simulink model "mpc_inertia_mass"  (R2022a)
settings: Solver=daessc  StartTime=0.0  StopTime=simlength  FixedStep=tcontrol  MaxStep=ts  RelTol=1e-3
undefined symbols (not defined in the file): Ad, Aled, Bd, Bled, C, Cle, Fmpc, Gmpc, Kd, Kmpc, Lled, load_torque, simlength, tc, tcontrol
libraries: nesl_utility x17, fl_lib x12, mass_spring_mass_lib x3
settings Model: SimulationMode=accelerator  Creator=dbagn  LastModifiedBy=dabagnara
settings SolverCC: AlgebraicLoopSolver=TrustRegion
settings DataIOCC: ReturnWorkspaceOutputs=off
settings DebuggingCC: UnconnectedInputMsg=warning  UnconnectedOutputMsg=warning  UnconnectedLineMsg=warning  SFMachineParentedDataDiag=warning
settings RTWCC: DLArmComputeVersion=19.05

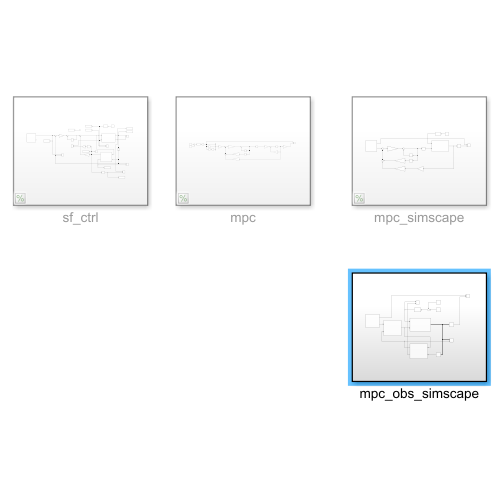
[thumbnail: Simulink's stored preview of the top-level diagram]
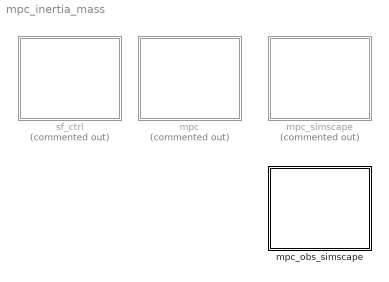
== system mpc_inertia_mass ==
  mpc : Subsystem  Commented=on
  mpc_obs_simscape : Subsystem
  mpc_simscape : Subsystem  Commented=on
  sf_ctrl : Subsystem  Commented=on

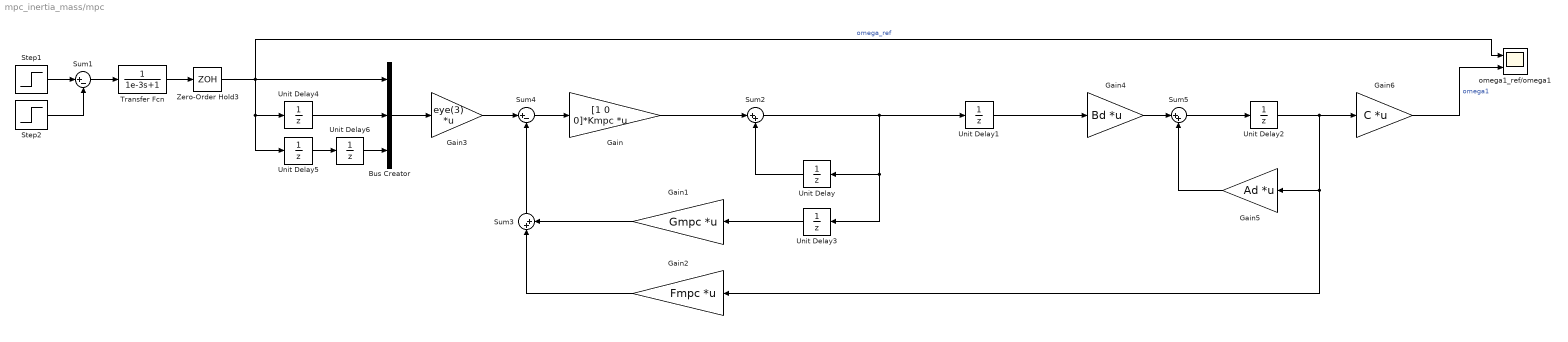
== system mpc_inertia_mass/mpc ==
  Bus Creator : BusCreator  Inputs=3
  Gain : Gain  Gain=[1 0 0]*Kmpc  Multiplication=Matrix(K*u)
  Gain1 : Gain  Gain=Gmpc  Multiplication=Matrix(K*u)
  Gain2 : Gain  Gain=Fmpc  Multiplication=Matrix(K*u)
  Gain3 : Gain  Gain=eye(3)  Multiplication=Matrix(K*u)
  Gain4 : Gain  Gain=Bd  Multiplication=Matrix(K*u)
  Gain5 : Gain  Gain=Ad  Multiplication=Matrix(K*u)
  Gain6 : Gain  Gain=C  Multiplication=Matrix(K*u)
  Step1 : Step  Time=0.2  SampleTime=0
  Step2 : Step  Time=simlength/2  SampleTime=0
  Sum1 : Sum  Inputs=|+-
  Sum2 : Sum  Inputs=|++
  Sum3 : Sum  Inputs=|++
  Sum4 : Sum  Inputs=|+-
  Sum5 : Sum  Inputs=|++
  Transfer Fcn : TransferFcn  Denominator=[1e-3 1]
  Unit Delay{,1..6} (7 alike) : UnitDelay  SampleTime=tcontrol  HasFrameUpgradeWarning=on
  Zero-Order Hold3 : ZeroOrderHold  SampleTime=tcontrol
  omega1_ref/omega1 : Scope  NumInputPorts=2
  wires:
  Step1/1 -> Sum1/1
  Step2/1 -> Sum1/2
  Gain/1 -> Sum2/1
  Unit Delay/1 -> Sum2/2
  Sum4/1 -> Gain/1
  Gain1/1 -> Sum3/2
  Sum3/1 -> Sum4/2
  Gain2/1 -> Sum3/1
  Gain4/1 -> Sum5/1
  Sum5/1 -> Unit Delay2/1
  Gain5/1 -> Sum5/2
  Gain6/1 -> omega1_ref/omega1/2  "omega1"
  Sum1/1 -> Transfer Fcn/1
  Transfer Fcn/1 -> Zero-Order Hold3/1
  Unit Delay3/1 -> Gain1/1
  Unit Delay2/1 -> Gain6/1, Gain2/1, Gain5/1
  Unit Delay5/1 -> Unit Delay6/1
  Unit Delay6/1 -> Bus Creator/3
  Unit Delay4/1 -> Bus Creator/2
  Zero-Order Hold3/1 -> Bus Creator/1, omega1_ref/omega1/1, Unit Delay5/1, Unit Delay4/1  "omega_ref"
  Bus Creator/1 -> Gain3/1
  Gain3/1 -> Sum4/1
  Sum2/1 -> Unit Delay1/1, Unit Delay3/1, Unit Delay/1
  Unit Delay1/1 -> Gain4/1

== system mpc_inertia_mass/mpc_obs_simscape ==
  Load_step : Step  Time=simlength/3  After=load_torque  SampleTime=0
  Load_step1 : Step  Time=2*simlength/3  After=-2*load_torque  SampleTime=0
  Selector : Selector  InputPortWidth=3  IndexOptions=Index vector (dialog)  Indices=[1 2]  OutputSizes=1
  Selector1 : Selector  InputPortWidth=3  IndexOptions=Index vector (dialog)  Indices=1  OutputSizes=1
  Sum : Sum  Inputs=++|
  Transfer Fcn : TransferFcn  Denominator=[1e-1 1]
  mpc : Subsystem
  observer td : Subsystem
  omega1_ref/omega1 : Scope  NumInputPorts=2
  omega1_ref/omega2 : Scope  NumInputPorts=2
  rference generator : Subsystem
  "simscape_plant " : Subsystem
  tau2/tau2_hat : Scope  NumInputPorts=2
  wires:
  Transfer Fcn/1 -> tau2/tau2_hat/1, "simscape_plant "/1(tau2)  "tau_2_flt"
  rference generator/1(omega_ref) -> omega1_ref/omega1/1
  "simscape_plant "/1(state) -> omega1_ref/omega2/1, Selector1/1, Selector/1  "omega1"
  Selector/1 -> omega1_ref/omega1/2  "omega12"
  Selector1/1 -> observer td/2(y)
  observer td/1(x_hat) -> omega1_ref/omega2/2, mpc/2(x_hat)
  observer td/2(tau2_hat) -> tau2/tau2_hat/2
  mpc/1(tau1) -> "simscape_plant "/2(tau1), observer td/1(u)
  rference generator/2(omega_ref_stack) -> mpc/1(yref)
  Load_step/1 -> Sum/2  "tau_2"
  Sum/1 -> Transfer Fcn/1
  Load_step1/1 -> Sum/1  "tau_2"

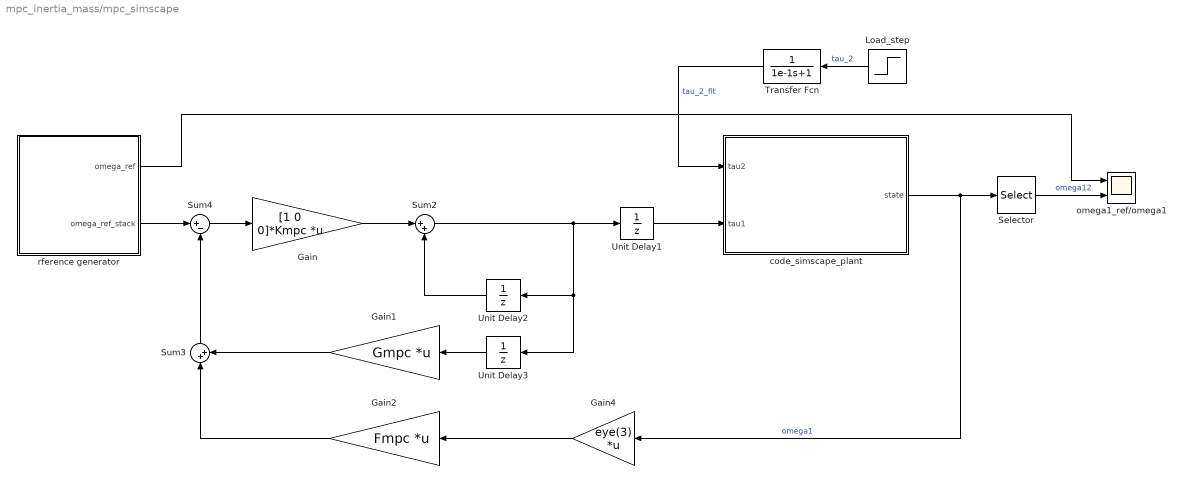
== system mpc_inertia_mass/mpc_simscape ==
  Gain : Gain  Gain=[1 0 0]*Kmpc  Multiplication=Matrix(K*u)
  Gain1 : Gain  Gain=Gmpc  Multiplication=Matrix(K*u)
  Gain2 : Gain  Gain=Fmpc  Multiplication=Matrix(K*u)
  Gain4 : Gain  Gain=eye(3)  Multiplication=Matrix(K*u)
  Load_step : Step  Time=simlength/3  After=load_torque  SampleTime=0
  Selector : Selector  InputPortWidth=3  IndexOptions=Index vector (dialog)  Indices=[1 2]  OutputSizes=1
  Sum2 : Sum  Inputs=|++
  Sum3 : Sum  Inputs=|++
  Sum4 : Sum  Inputs=|+-
  Transfer Fcn : TransferFcn  Denominator=[1e-1 1]
  Unit Delay1 : UnitDelay  SampleTime=tcontrol  HasFrameUpgradeWarning=on
  Unit Delay2 : UnitDelay  SampleTime=tcontrol  HasFrameUpgradeWarning=on
  Unit Delay3 : UnitDelay  SampleTime=tcontrol  HasFrameUpgradeWarning=on
  "code_simscape_plant " : Subsystem
  omega1_ref/omega1 : Scope  NumInputPorts=2
  rference generator : Subsystem
  wires:
  Selector/1 -> omega1_ref/omega1/2  "omega12"
  Gain2/1 -> Sum3/1
  Sum3/1 -> Sum4/2
  Gain1/1 -> Sum3/2
  Sum4/1 -> Gain/1
  Gain/1 -> Sum2/1
  "code_simscape_plant "/1(state) -> Selector/1, Gain4/1  "omega1"
  Gain4/1 -> Gain2/1
  Unit Delay2/1 -> Sum2/2
  Unit Delay3/1 -> Gain1/1
  Sum2/1 -> Unit Delay1/1, Unit Delay3/1, Unit Delay2/1
  Unit Delay1/1 -> "code_simscape_plant "/2(tau1)
  rference generator/1(omega_ref) -> omega1_ref/omega1/1
  rference generator/2(omega_ref_stack) -> Sum4/1
  Load_step/1 -> Transfer Fcn/1  "tau_2"
  Transfer Fcn/1 -> "code_simscape_plant "/1(tau2)  "tau_2_flt"

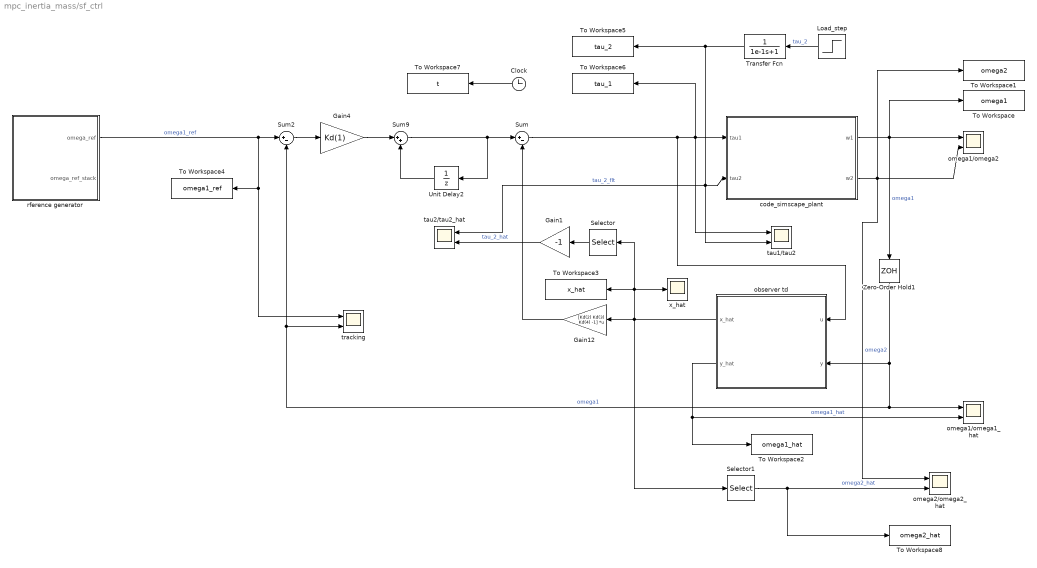
== system mpc_inertia_mass/sf_ctrl ==
  Clock : Clock
  Gain1 : Gain  Gain=-1
  Gain12 : Gain  Gain=[Kd(2) Kd(3) Kd(4) -1]  Multiplication=Matrix(K*u)
  Gain4 : Gain  Gain=Kd(1)
  Load_step : Step  Time=simlength/3  After=load_torque  SampleTime=0
  Selector : Selector  InputPortWidth=4  IndexOptions=Index vector (dialog)  Indices=4  OutputSizes=1
  Selector1 : Selector  InputPortWidth=4  IndexOptions=Index vector (dialog)  Indices=2  OutputSizes=1
  Sum : Sum  Inputs=|+-
  Sum2 : Sum  Inputs=|+-
  Sum9 : Sum  Inputs=|++
  To Workspace : ToWorkspace  VariableName=omega1  SampleTime=tc
      settings: MaxDataPoints=Nc
  To Workspace1 : ToWorkspace  VariableName=omega2  SampleTime=tc
      settings: MaxDataPoints=Nc
  To Workspace2 : ToWorkspace  VariableName=omega1_hat  SampleTime=tc
      settings: MaxDataPoints=Nc
  To Workspace3 : ToWorkspace  VariableName=x_hat  SampleTime=tc
      settings: MaxDataPoints=Nc
  To Workspace4 : ToWorkspace  VariableName=omega1_ref  SampleTime=tc
      settings: MaxDataPoints=Nc
  To Workspace5 : ToWorkspace  VariableName=tau_2  SampleTime=tc
      settings: MaxDataPoints=Nc
  To Workspace6 : ToWorkspace  VariableName=tau_1  SampleTime=tc
      settings: MaxDataPoints=Nc
  To Workspace7 : ToWorkspace  VariableName=t  SampleTime=tc
      settings: MaxDataPoints=Nc
  To Workspace8 : ToWorkspace  VariableName=omega2_hat  SampleTime=tc
      settings: MaxDataPoints=Nc
  Transfer Fcn : TransferFcn  Denominator=[1e-1 1]
  Unit Delay2 : UnitDelay  SampleTime=tcontrol  HasFrameUpgradeWarning=on
  Zero-Order Hold1 : ZeroOrderHold  SampleTime=tcontrol
  "code_simscape_plant " : Subsystem
  observer td : Subsystem
  omega1/omega1_hat : Scope  NumInputPorts=2
  omega1/omega2 : Scope  NumInputPorts=2
  omega2/omega2_hat : Scope  NumInputPorts=2
  rference generator : Subsystem
  tau1/tau2 : Scope  NumInputPorts=2
  tau2/tau2_hat : Scope  NumInputPorts=2
  tracking : Scope  NumInputPorts=2
  x_hat : Scope
  wires:
  Sum9/1 -> Sum/1, Unit Delay2/1
  Transfer Fcn/1 -> To Workspace5/1, "code_simscape_plant "/2(tau2), tau1/tau2/2, tau2/tau2_hat/1  "tau_2_flt"
  observer td/1(x_hat) -> Selector1/1, Selector/1, To Workspace3/1, x_hat/1, Gain12/1
  Selector1/1 -> To Workspace8/1, omega2/omega2_hat/2  "omega2_hat"
  Gain12/1 -> Sum/2
  "code_simscape_plant "/2(w2) -> To Workspace1/1, omega1/omega2/2, omega2/omega2_hat/1  "omega2"
  "code_simscape_plant "/1(w1) -> Zero-Order Hold1/1, To Workspace/1, omega1/omega2/1  "omega1"
  Gain4/1 -> Sum9/1
  Zero-Order Hold1/1 -> tracking/2, Sum2/2, omega1/omega1_hat/1, observer td/2(y)  "omega1"
  Load_step/1 -> Transfer Fcn/1  "tau_2"
  observer td/2(y_hat) -> To Workspace2/1, omega1/omega1_hat/2  "omega1_hat"
  rference generator/1(omega_ref) -> To Workspace4/1, tracking/1, Sum2/1  "omega1_ref"
  Gain1/1 -> tau2/tau2_hat/2  "tau_2_hat"
  Clock/1 -> To Workspace7/1
  Sum2/1 -> Gain4/1
  Selector/1 -> Gain1/1
  Unit Delay2/1 -> Sum9/2
  Sum/1 -> tau1/tau2/1, "code_simscape_plant "/1(tau1), To Workspace6/1, observer td/1(u)

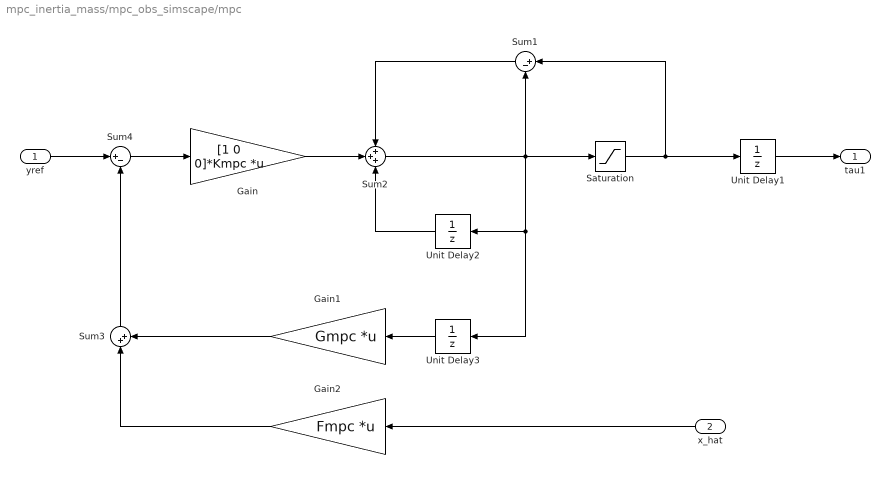
== system mpc_inertia_mass/mpc_obs_simscape/mpc ==
  yref : Inport
  x_hat : Inport  Port=2
  Gain : Gain  Gain=[1 0 0]*Kmpc  Multiplication=Matrix(K*u)
  Gain1 : Gain  Gain=Gmpc  Multiplication=Matrix(K*u)
  Gain2 : Gain  Gain=Fmpc  Multiplication=Matrix(K*u)
  Saturation : Saturate  UpperLimit=2000  LowerLimit=-2000
  Sum1 : Sum  Inputs=|+-
  Sum2 : Sum  Inputs=+++
  Sum3 : Sum  Inputs=|++
  Sum4 : Sum  Inputs=|+-
  Unit Delay1 : UnitDelay  SampleTime=tcontrol  HasFrameUpgradeWarning=on
  Unit Delay2 : UnitDelay  SampleTime=tcontrol  HasFrameUpgradeWarning=on
  Unit Delay3 : UnitDelay  SampleTime=tcontrol  HasFrameUpgradeWarning=on
  tau1 : Outport
  wires:
  Sum3/1 -> Sum4/2
  Gain1/1 -> Sum3/2
  Sum4/1 -> Gain/1
  Gain2/1 -> Sum3/1
  x_hat/1 -> Gain2/1
  Unit Delay3/1 -> Gain1/1
  yref/1 -> Sum4/1
  Sum2/1 -> Sum1/2, Saturation/1, Unit Delay2/1, Unit Delay3/1
  Gain/1 -> Sum2/2
  Unit Delay2/1 -> Sum2/3
  Sum1/1 -> Sum2/1
  Saturation/1 -> Unit Delay1/1, Sum1/1
  Unit Delay1/1 -> tau1/1

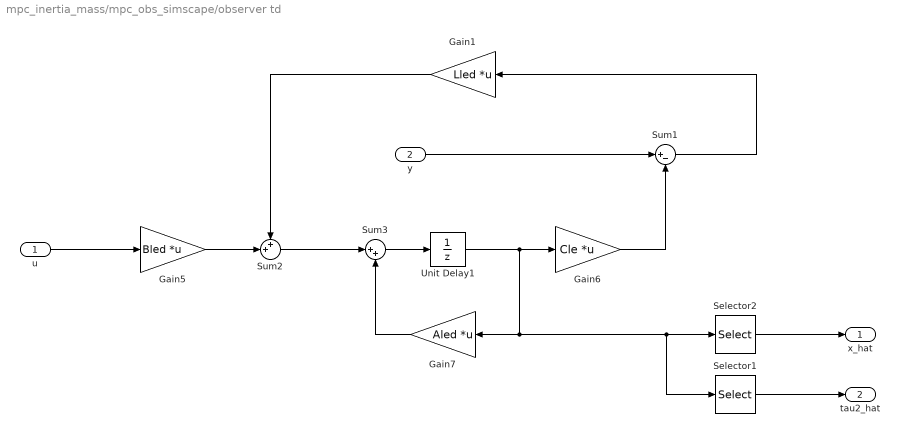
== system mpc_inertia_mass/mpc_obs_simscape/observer td ==
  u : Inport
  y : Inport  Port=2
  Gain1 : Gain  Gain=Lled  Multiplication=Matrix(K*u)
  Gain5 : Gain  Gain=Bled  Multiplication=Matrix(K*u)
  Gain6 : Gain  Gain=Cle  Multiplication=Matrix(K*u)
  Gain7 : Gain  Gain=Aled  Multiplication=Matrix(K*u)
  Selector1 : Selector  InputPortWidth=4  IndexOptions=Index vector (dialog)  Indices=4  OutputSizes=1
  Selector2 : Selector  InputPortWidth=4  IndexOptions=Index vector (dialog)  Indices=[1 2 3]  OutputSizes=1
  Sum1 : Sum  Inputs=|+-
  Sum2 : Sum  Inputs=++|
  Sum3 : Sum  Inputs=|++
  Unit Delay1 : UnitDelay  SampleTime=tcontrol  HasFrameUpgradeWarning=on
  x_hat : Outport
  tau2_hat : Outport  Port=2
  wires:
  Sum2/1 -> Sum3/1
  Sum3/1 -> Unit Delay1/1
  Gain7/1 -> Sum3/2
  Gain6/1 -> Sum1/2
  Sum1/1 -> Gain1/1
  u/1 -> Gain5/1
  Gain1/1 -> Sum2/1
  Gain5/1 -> Sum2/2
  Unit Delay1/1 -> Selector1/1, Selector2/1, Gain7/1, Gain6/1
  y/1 -> Sum1/1
  Selector2/1 -> x_hat/1
  Selector1/1 -> tau2_hat/1

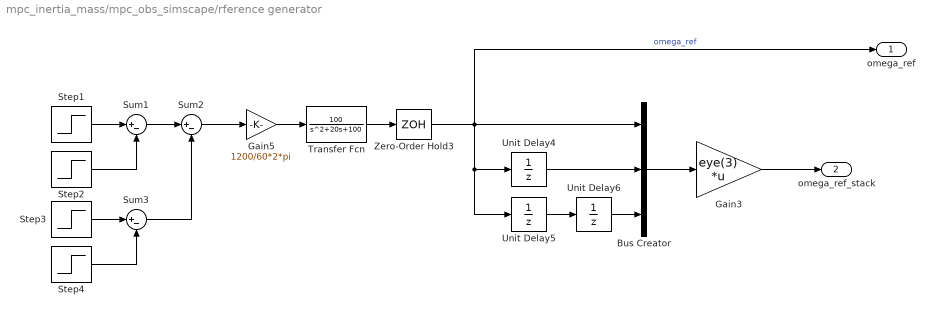
== system mpc_inertia_mass/mpc_obs_simscape/rference generator ==
  Bus Creator : BusCreator  Inputs=3
  Gain3 : Gain  Gain=eye(3)  Multiplication=Matrix(K*u)
  Gain5 : Gain  Gain=1200/60*2*pi
  Step1 : Step  Time=2  SampleTime=0
  Step2 : Step  Time=simlength/4  SampleTime=0
  Step3 : Step  Time=simlength/2  SampleTime=0
  Step4 : Step  Time=2*simlength/3  SampleTime=0
  Sum1 : Sum  Inputs=|+-
  Sum2 : Sum  Inputs=|+-
  Sum3 : Sum  Inputs=|+-
  Transfer Fcn : TransferFcn  Numerator=[100]  Denominator=[1 20 100]
  Unit Delay4 : UnitDelay  SampleTime=tcontrol  HasFrameUpgradeWarning=on
  Unit Delay5 : UnitDelay  SampleTime=tcontrol  HasFrameUpgradeWarning=on
  Unit Delay6 : UnitDelay  SampleTime=tcontrol  HasFrameUpgradeWarning=on
  Zero-Order Hold3 : ZeroOrderHold  SampleTime=tcontrol
  omega_ref : Outport
  omega_ref_stack : Outport  Port=2
  wires:
  Sum3/1 -> Sum2/2
  Step4/1 -> Sum3/2
  Step3/1 -> Sum3/1
  Sum2/1 -> Gain5/1
  Sum1/1 -> Sum2/1
  Gain3/1 -> omega_ref_stack/1
  Step1/1 -> Sum1/1
  Transfer Fcn/1 -> Zero-Order Hold3/1
  Step2/1 -> Sum1/2
  Unit Delay5/1 -> Unit Delay6/1
  Unit Delay6/1 -> Bus Creator/3
  Zero-Order Hold3/1 -> Bus Creator/1, Unit Delay5/1, Unit Delay4/1, omega_ref/1  "omega_ref"
  Bus Creator/1 -> Gain3/1
  Gain5/1 -> Transfer Fcn/1
  Unit Delay4/1 -> Bus Creator/2

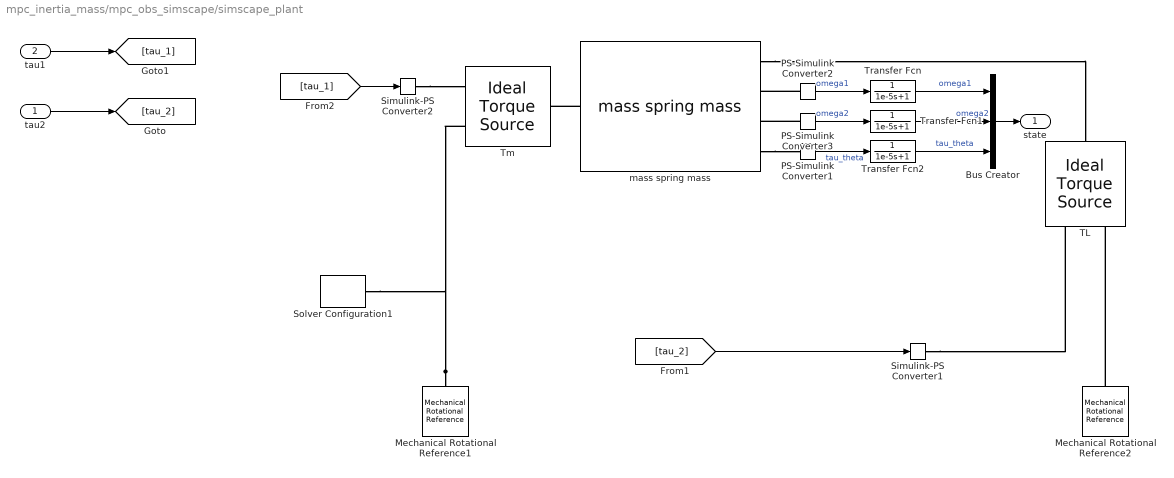
== system mpc_inertia_mass/mpc_obs_simscape/simscape_plant  ==
  tau2 : Inport
  tau1 : Inport  Port=2
  Bus Creator : BusCreator  Inputs=3
  Mechanical Rotational Reference1 : fl_lib/Mechanical/Rotational Elements/Mechanical Rotational Reference
      settings: SourceProductBaseCode=PW,SS,VE
  Mechanical Rotational Reference2 : fl_lib/Mechanical/Rotational Elements/Mechanical Rotational Reference
      settings: SourceProductBaseCode=PW,SS,VE
  PS-Simulink Converter1 : nesl_utility/PS-Simulink Converter  PhysicalDomain=network_engine_domain  SubClassName=ps_output  LeftPortType=input  RightPortType=output  PseudoPeriodic=off  Frequencies=[]  VectorFormat=1-D array  Unit=N*m  AffineConversion=on
      settings: SourceProductBaseCode=SS,PW,VE
  PS-Simulink Converter2 : nesl_utility/PS-Simulink Converter  PhysicalDomain=network_engine_domain  SubClassName=ps_output  LeftPortType=input  RightPortType=output  PseudoPeriodic=off  Frequencies=[]  VectorFormat=1-D array  Unit=rad/s  AffineConversion=on
      settings: SourceProductBaseCode=SS,PW,VE
  PS-Simulink Converter3 : nesl_utility/PS-Simulink Converter  PhysicalDomain=network_engine_domain  SubClassName=ps_output  LeftPortType=input  RightPortType=output  PseudoPeriodic=off  Frequencies=[]  VectorFormat=1-D array  Unit=rad/s  AffineConversion=on
      settings: SourceProductBaseCode=SS,PW,VE
  Simulink-PS Converter1 : nesl_utility/Simulink-PS Converter  PhysicalDomain=network_engine_domain  SubClassName=ps_input  LeftPortType=input  RightPortType=output  PseudoPeriodic=off  Frequencies=[]  NoiseDistribution=none  NoiseParameters=[]  Unit=1  AffineConversion=off  FilteringAndDerivatives=provide  SimscapeFilterOrder=1  InputFilterTimeConstant=0.001  UdotUserProvided=0
      settings: SourceProductBaseCode=SS,PW,VE
  Simulink-PS Converter2 : nesl_utility/Simulink-PS Converter  PhysicalDomain=network_engine_domain  SubClassName=ps_input  LeftPortType=input  RightPortType=output  PseudoPeriodic=off  Frequencies=[]  NoiseDistribution=none  NoiseParameters=[]  Unit=1  AffineConversion=off  FilteringAndDerivatives=provide  SimscapeFilterOrder=1  InputFilterTimeConstant=0.001  UdotUserProvided=0
      settings: SourceProductBaseCode=SS,PW,VE
  Solver Configuration1 : nesl_utility/Solver Configuration  PhysicalDomain=network_engine_domain  SubClassName=solver  LeftPortType=input  RightPortType=generic  Tones=[]  Harmonics=[]  SimulateNoise=off  Profile=off  UseLocalSampling=off  EnableSwitchedLinearOptims=on  FrequencyDomain=off  UseCCode=off  RelTol=0.001  AbsTol=1e-06  MinStep=1e-09  ToWorkspace=off  RevertToSquareIcSolve=off  NumHomotopyIterations=100  PhasorMode=off  PhasorModeNumHarmonics=1  IndexReductionMethod=DerivativeReplacement  DoDC=off  ResidualTolerance=1e-09  UseLocalSolver=on  LocalSolverChoice=NE_BACKWARD_EULER_ADVANCER  LocalSolverSampleTime=ts  DoFixedCost=on  MaxNonlinIter=3  MaxModeIter=2  ComputeImpulses=off  ImpulseIterations=2  LinearAlgebra=auto  LinearAlgebraNumThread=0  EquationFormulation=NE_TIME_EF  DelaysMemoryBudget=1024  AutomaticFiltering=on  FilteringTimeConstant=0.001  PartitionStorageMethod=AS_NEEDED  PartitionMemoryBudget=1024  PartitionMethod=ROBUST
      settings: SourceProductBaseCode=SS,PW,VE
  TL : fl_lib/Mechanical/Mechanical Sources/Ideal Torque Source
      settings: SourceProductBaseCode=PW,SS,VE
  "Tm " : fl_lib/Mechanical/Mechanical Sources/Ideal Torque Source
      settings: SourceProductBaseCode=PW,SS,VE
  Transfer Fcn : TransferFcn  Denominator=[1e-5 1]
  Transfer Fcn1 : TransferFcn  Denominator=[1e-5 1]
  Transfer Fcn2 : TransferFcn  Denominator=[1e-5 1]
  mass spring mass : mass_spring_mass_lib/mass spring mass  b1=b N*m/(rad/s)  J1=J1 kg*m^2  b2=b N*m/(rad/s)  J2=J2 kg*m^2  b_theta=b_theta N*m/(rad/s)  k_theta=k_theta N*m/rad  omega_1_specify=off  omega_1_priority=None  omega_1=0 rad/s  omega_1_nominal_specify=off  omega_1_nominal_unit=rad/s  omega_1_nominal_value=1  omega_2_specify=off  omega_2_priority=None  omega_2=0 rad/s  omega_2_nominal_specify=off  omega_2_nominal_unit=rad/s  omega_2_nominal_value=1  tau_1_specify=off  tau_1_priority=None  tau_1=0 N*m  tau_1_nominal_specify=off  tau_1_nominal_unit=N*m  tau_1_nominal_value=1  tau_2_specify=off  tau_2_priority=None  tau_2=0 N*m  tau_2_nominal_specify=off  tau_2_nominal_unit=N*m  tau_2_nominal_value=1  tau_theta_specify=off  tau_theta_priority=None  tau_theta=0 N*m  tau_theta_nominal_specify=off  tau_theta_nominal_unit=N*m  tau_theta_nominal_value=1
      settings: InternalSimscapePortConfiguration="{\"Bottom\":[],\"Left\":[{\"id\":\"S1\",\"label\":\"S1\",\"type\":\"foundation.mechanical.rotational.rotational\"}],\"Right\":[{\"id\":\"S2\",\"label\":\"S2\",\"type\":\"foundation.mechanical.rotational.rotational\"},{\"id\":\"omega1_out\",\"label\":\"omega1\",\"type\":\"output\"},{\"id\":\"omega2_out\",\"label\":\"omega2\",\"type\":\"output\"},{\"id\":\"tau_theta_out\",\"label\":\"tau_theta\",\"type\":\"output\"}],\"Top\":[]}"
  state : Outport
  wires:
  Transfer Fcn2/1 -> Bus Creator/3  "tau_theta"
  Transfer Fcn1/1 -> Bus Creator/2  "omega2"
  Transfer Fcn/1 -> Bus Creator/1  "omega1"
  PS-Simulink Converter1/1 -> Transfer Fcn2/1  "tau_theta"
  PS-Simulink Converter3/1 -> Transfer Fcn1/1  "omega2"
  PS-Simulink Converter2/1 -> Transfer Fcn/1  "omega1"
  tau2/1 -> [tau_2]
  [tau_1] -> Simulink-PS Converter2/1
  tau1/1 -> [tau_1]
  [tau_2] -> Simulink-PS Converter1/1
  Bus Creator/1 -> state/1
  connections:
  Mechanical Rotational Reference2/LConn1 -- TL/RConn2
  Mechanical Rotational Reference1/LConn1 -- "Tm "/RConn2 -- Solver Configuration1/RConn1
  mass spring mass/RConn1 -- TL/LConn1
  Simulink-PS Converter1/RConn1 -- TL/RConn1
  mass spring mass/LConn1 -- "Tm "/LConn1
  Simulink-PS Converter2/RConn1 -- "Tm "/RConn1
  mass spring mass/RConn4 -- PS-Simulink Converter1/LConn1
  PS-Simulink Converter3/LConn1 -- mass spring mass/RConn3
  PS-Simulink Converter2/LConn1 -- mass spring mass/RConn2

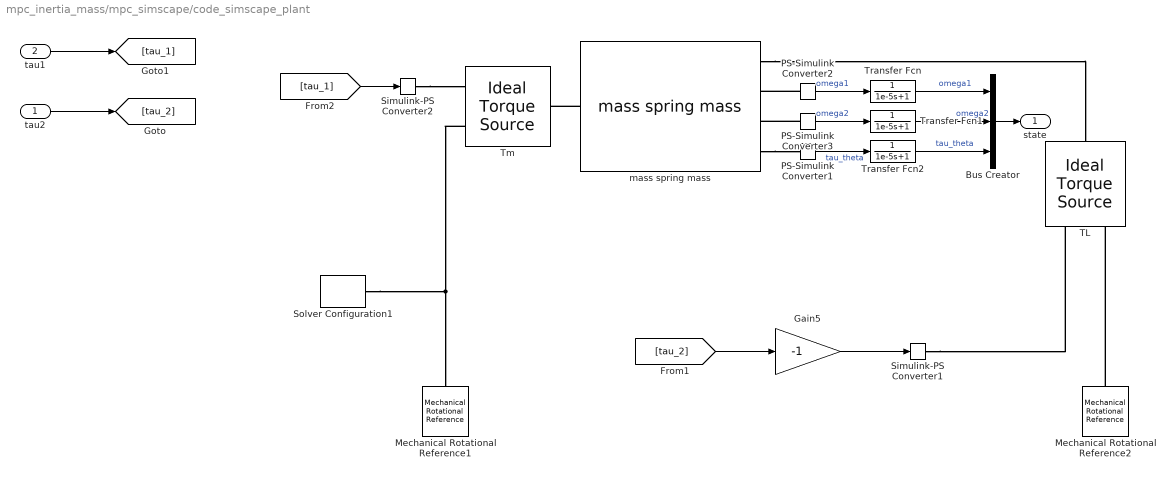
== system mpc_inertia_mass/mpc_simscape/code_simscape_plant  ==
  tau2 : Inport
  tau1 : Inport  Port=2
  Bus Creator : BusCreator  Inputs=3
  Gain5 : Gain  Gain=-1
  Mechanical Rotational Reference1 : fl_lib/Mechanical/Rotational Elements/Mechanical Rotational Reference
      settings: SourceProductBaseCode=PW,SS,VE
  Mechanical Rotational Reference2 : fl_lib/Mechanical/Rotational Elements/Mechanical Rotational Reference
      settings: SourceProductBaseCode=PW,SS,VE
  PS-Simulink Converter1 : nesl_utility/PS-Simulink Converter  PhysicalDomain=network_engine_domain  SubClassName=ps_output  LeftPortType=input  RightPortType=output  PseudoPeriodic=off  Frequencies=[]  VectorFormat=1-D array  Unit=N*m  AffineConversion=on
      settings: SourceProductBaseCode=SS,PW,VE
  PS-Simulink Converter2 : nesl_utility/PS-Simulink Converter  PhysicalDomain=network_engine_domain  SubClassName=ps_output  LeftPortType=input  RightPortType=output  PseudoPeriodic=off  Frequencies=[]  VectorFormat=1-D array  Unit=rad/s  AffineConversion=on
      settings: SourceProductBaseCode=SS,PW,VE
  PS-Simulink Converter3 : nesl_utility/PS-Simulink Converter  PhysicalDomain=network_engine_domain  SubClassName=ps_output  LeftPortType=input  RightPortType=output  PseudoPeriodic=off  Frequencies=[]  VectorFormat=1-D array  Unit=rad/s  AffineConversion=on
      settings: SourceProductBaseCode=SS,PW,VE
  Simulink-PS Converter1 : nesl_utility/Simulink-PS Converter  PhysicalDomain=network_engine_domain  SubClassName=ps_input  LeftPortType=input  RightPortType=output  PseudoPeriodic=off  Frequencies=[]  NoiseDistribution=none  NoiseParameters=[]  Unit=1  AffineConversion=off  FilteringAndDerivatives=provide  SimscapeFilterOrder=1  InputFilterTimeConstant=0.001  UdotUserProvided=0
      settings: SourceProductBaseCode=SS,PW,VE
  Simulink-PS Converter2 : nesl_utility/Simulink-PS Converter  PhysicalDomain=network_engine_domain  SubClassName=ps_input  LeftPortType=input  RightPortType=output  PseudoPeriodic=off  Frequencies=[]  NoiseDistribution=none  NoiseParameters=[]  Unit=1  AffineConversion=off  FilteringAndDerivatives=provide  SimscapeFilterOrder=1  InputFilterTimeConstant=0.001  UdotUserProvided=0
      settings: SourceProductBaseCode=SS,PW,VE
  Solver Configuration1 : nesl_utility/Solver Configuration  PhysicalDomain=network_engine_domain  SubClassName=solver  LeftPortType=input  RightPortType=generic  Tones=[]  Harmonics=[]  SimulateNoise=off  Profile=off  UseLocalSampling=off  EnableSwitchedLinearOptims=on  FrequencyDomain=off  UseCCode=off  RelTol=0.001  AbsTol=1e-06  MinStep=1e-09  ToWorkspace=off  RevertToSquareIcSolve=off  NumHomotopyIterations=100  PhasorMode=off  PhasorModeNumHarmonics=1  IndexReductionMethod=DerivativeReplacement  DoDC=off  ResidualTolerance=1e-09  UseLocalSolver=on  LocalSolverChoice=NE_TRAPEZOIDAL_ADVANCER  LocalSolverSampleTime=ts  DoFixedCost=on  MaxNonlinIter=3  MaxModeIter=2  ComputeImpulses=off  ImpulseIterations=2  LinearAlgebra=auto  LinearAlgebraNumThread=0  EquationFormulation=NE_TIME_EF  DelaysMemoryBudget=1024  AutomaticFiltering=on  FilteringTimeConstant=0.001  PartitionStorageMethod=AS_NEEDED  PartitionMemoryBudget=1024  PartitionMethod=ROBUST
      settings: SourceProductBaseCode=SS,PW,VE
  TL : fl_lib/Mechanical/Mechanical Sources/Ideal Torque Source
      settings: SourceProductBaseCode=PW,SS,VE
  "Tm " : fl_lib/Mechanical/Mechanical Sources/Ideal Torque Source
      settings: SourceProductBaseCode=PW,SS,VE
  Transfer Fcn : TransferFcn  Denominator=[1e-5 1]
  Transfer Fcn1 : TransferFcn  Denominator=[1e-5 1]
  Transfer Fcn2 : TransferFcn  Denominator=[1e-5 1]
  mass spring mass : mass_spring_mass_lib/mass spring mass  b1=b N*m/(rad/s)  J1=J1 kg*m^2  b2=b N*m/(rad/s)  J2=J2 kg*m^2  b_theta=b_theta N*m/(rad/s)  k_theta=k_theta N*m/rad  omega_1_specify=off  omega_1_priority=None  omega_1=0 rad/s  omega_1_nominal_specify=off  omega_1_nominal_unit=rad/s  omega_1_nominal_value=1  omega_2_specify=off  omega_2_priority=None  omega_2=0 rad/s  omega_2_nominal_specify=off  omega_2_nominal_unit=rad/s  omega_2_nominal_value=1  tau_1_specify=off  tau_1_priority=None  tau_1=0 N*m  tau_1_nominal_specify=off  tau_1_nominal_unit=N*m  tau_1_nominal_value=1  tau_2_specify=off  tau_2_priority=None  tau_2=0 N*m  tau_2_nominal_specify=off  tau_2_nominal_unit=N*m  tau_2_nominal_value=1  tau_theta_specify=off  tau_theta_priority=None  tau_theta=0 N*m  tau_theta_nominal_specify=off  tau_theta_nominal_unit=N*m  tau_theta_nominal_value=1
      settings: InternalSimscapePortConfiguration="{\"Bottom\":[],\"Left\":[{\"id\":\"S1\",\"label\":\"S1\",\"type\":\"foundation.mechanical.rotational.rotational\"}],\"Right\":[{\"id\":\"S2\",\"label\":\"S2\",\"type\":\"foundation.mechanical.rotational.rotational\"},{\"id\":\"omega1_out\",\"label\":\"omega1\",\"type\":\"output\"},{\"id\":\"omega2_out\",\"label\":\"omega2\",\"type\":\"output\"},{\"id\":\"tau_theta_out\",\"label\":\"tau_theta\",\"type\":\"output\"}],\"Top\":[]}"
  state : Outport
  wires:
  Bus Creator/1 -> state/1
  Gain5/1 -> Simulink-PS Converter1/1
  tau1/1 -> [tau_1]
  [tau_1] -> Simulink-PS Converter2/1
  tau2/1 -> [tau_2]
  [tau_2] -> Gain5/1
  PS-Simulink Converter2/1 -> Transfer Fcn/1  "omega1"
  PS-Simulink Converter3/1 -> Transfer Fcn1/1  "omega2"
  PS-Simulink Converter1/1 -> Transfer Fcn2/1  "tau_theta"
  Transfer Fcn/1 -> Bus Creator/1  "omega1"
  Transfer Fcn1/1 -> Bus Creator/2  "omega2"
  Transfer Fcn2/1 -> Bus Creator/3  "tau_theta"
  connections:
  PS-Simulink Converter2/LConn1 -- mass spring mass/RConn2
  PS-Simulink Converter3/LConn1 -- mass spring mass/RConn3
  mass spring mass/RConn4 -- PS-Simulink Converter1/LConn1
  Simulink-PS Converter2/RConn1 -- "Tm "/RConn1
  mass spring mass/LConn1 -- "Tm "/LConn1
  Simulink-PS Converter1/RConn1 -- TL/RConn1
  mass spring mass/RConn1 -- TL/LConn1
  Solver Configuration1/RConn1 -- "Tm "/RConn2 -- Mechanical Rotational Reference1/LConn1
  Mechanical Rotational Reference2/LConn1 -- TL/RConn2

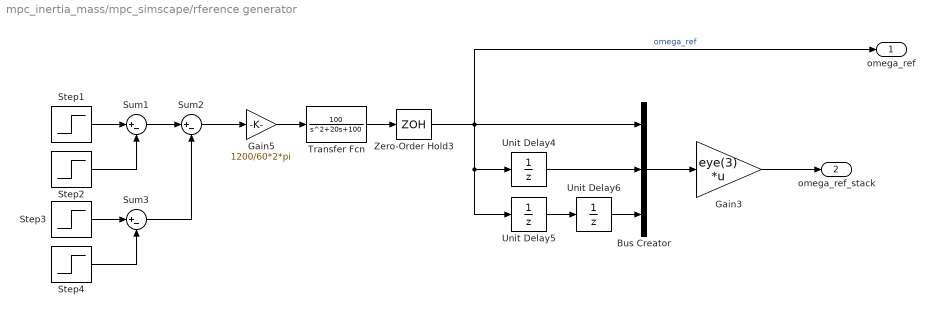
== system mpc_inertia_mass/mpc_simscape/rference generator ==
  Bus Creator : BusCreator  Inputs=3
  Gain3 : Gain  Gain=eye(3)  Multiplication=Matrix(K*u)
  Gain5 : Gain  Gain=1200/60*2*pi
  Step1 : Step  Time=2  SampleTime=0
  Step2 : Step  Time=simlength/4  SampleTime=0
  Step3 : Step  Time=simlength/2  SampleTime=0
  Step4 : Step  Time=2*simlength/3  SampleTime=0
  Sum1 : Sum  Inputs=|+-
  Sum2 : Sum  Inputs=|+-
  Sum3 : Sum  Inputs=|+-
  Transfer Fcn : TransferFcn  Numerator=[100]  Denominator=[1 20 100]
  Unit Delay4 : UnitDelay  SampleTime=tcontrol  HasFrameUpgradeWarning=on
  Unit Delay5 : UnitDelay  SampleTime=tcontrol  HasFrameUpgradeWarning=on
  Unit Delay6 : UnitDelay  SampleTime=tcontrol  HasFrameUpgradeWarning=on
  Zero-Order Hold3 : ZeroOrderHold  SampleTime=tcontrol
  omega_ref : Outport
  omega_ref_stack : Outport  Port=2
  wires:
  Unit Delay4/1 -> Bus Creator/2
  Gain5/1 -> Transfer Fcn/1
  Bus Creator/1 -> Gain3/1
  Zero-Order Hold3/1 -> omega_ref/1, Unit Delay4/1, Unit Delay5/1, Bus Creator/1  "omega_ref"
  Unit Delay6/1 -> Bus Creator/3
  Unit Delay5/1 -> Unit Delay6/1
  Step2/1 -> Sum1/2
  Transfer Fcn/1 -> Zero-Order Hold3/1
  Step1/1 -> Sum1/1
  Gain3/1 -> omega_ref_stack/1
  Sum1/1 -> Sum2/1
  Sum2/1 -> Gain5/1
  Step3/1 -> Sum3/1
  Step4/1 -> Sum3/2
  Sum3/1 -> Sum2/2

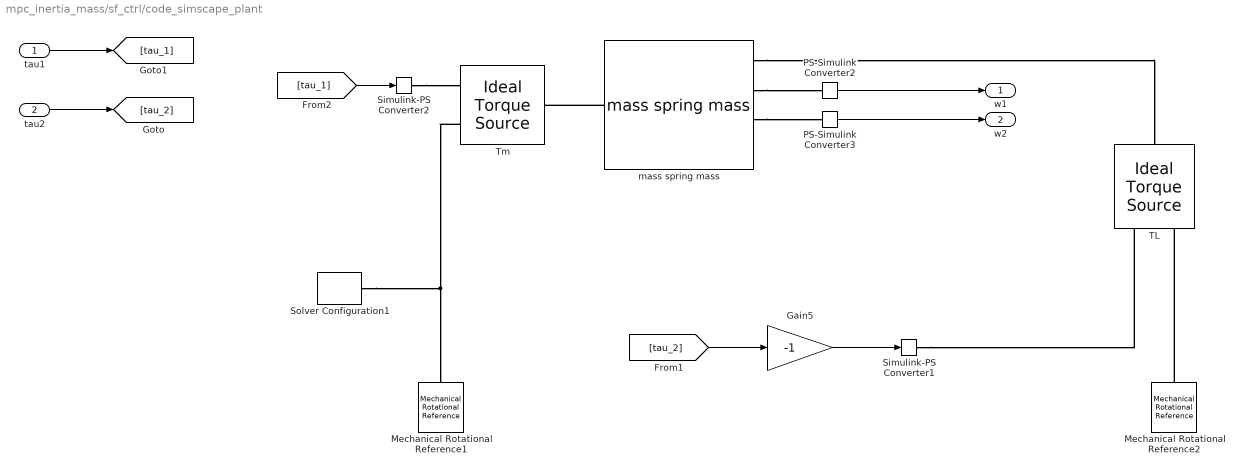
== system mpc_inertia_mass/sf_ctrl/code_simscape_plant  ==
  tau1 : Inport
  tau2 : Inport  Port=2
  Gain5 : Gain  Gain=-1
  Mechanical Rotational Reference1 : fl_lib/Mechanical/Rotational Elements/Mechanical Rotational Reference
      settings: SourceProductBaseCode=PW,SS,VE
  Mechanical Rotational Reference2 : fl_lib/Mechanical/Rotational Elements/Mechanical Rotational Reference
      settings: SourceProductBaseCode=PW,SS,VE
  PS-Simulink Converter2 : nesl_utility/PS-Simulink Converter  PhysicalDomain=network_engine_domain  SubClassName=ps_output  LeftPortType=input  RightPortType=output  PseudoPeriodic=off  Frequencies=[]  VectorFormat=1-D array  Unit=1  AffineConversion=off
      settings: SourceProductBaseCode=SS,PW,VE
  PS-Simulink Converter3 : nesl_utility/PS-Simulink Converter  PhysicalDomain=network_engine_domain  SubClassName=ps_output  LeftPortType=input  RightPortType=output  PseudoPeriodic=off  Frequencies=[]  VectorFormat=1-D array  Unit=1  AffineConversion=off
      settings: SourceProductBaseCode=SS,PW,VE
  Simulink-PS Converter1 : nesl_utility/Simulink-PS Converter  PhysicalDomain=network_engine_domain  SubClassName=ps_input  LeftPortType=input  RightPortType=output  PseudoPeriodic=off  Frequencies=[]  NoiseDistribution=none  NoiseParameters=[]  Unit=1  AffineConversion=off  FilteringAndDerivatives=provide  SimscapeFilterOrder=1  InputFilterTimeConstant=0.001  UdotUserProvided=0
      settings: SourceProductBaseCode=SS,PW,VE
  Simulink-PS Converter2 : nesl_utility/Simulink-PS Converter  PhysicalDomain=network_engine_domain  SubClassName=ps_input  LeftPortType=input  RightPortType=output  PseudoPeriodic=off  Frequencies=[]  NoiseDistribution=none  NoiseParameters=[]  Unit=1  AffineConversion=off  FilteringAndDerivatives=provide  SimscapeFilterOrder=1  InputFilterTimeConstant=0.001  UdotUserProvided=0
      settings: SourceProductBaseCode=SS,PW,VE
  Solver Configuration1 : nesl_utility/Solver Configuration  PhysicalDomain=network_engine_domain  SubClassName=solver  LeftPortType=input  RightPortType=generic  Tones=[]  Harmonics=[]  SimulateNoise=off  Profile=off  UseLocalSampling=off  EnableSwitchedLinearOptims=on  FrequencyDomain=off  UseCCode=off  RelTol=0.001  AbsTol=1e-06  MinStep=1e-09  ToWorkspace=off  RevertToSquareIcSolve=off  NumHomotopyIterations=100  PhasorMode=off  PhasorModeNumHarmonics=1  IndexReductionMethod=DerivativeReplacement  DoDC=off  ResidualTolerance=1e-09  UseLocalSolver=off  LocalSolverChoice=NE_TRAPEZOIDAL_ADVANCER  LocalSolverSampleTime=ts  DoFixedCost=off  MaxNonlinIter=3  MaxModeIter=2  ComputeImpulses=off  ImpulseIterations=2  LinearAlgebra=auto  LinearAlgebraNumThread=0  EquationFormulation=NE_TIME_EF  DelaysMemoryBudget=1024  AutomaticFiltering=on  FilteringTimeConstant=0.001  PartitionStorageMethod=AS_NEEDED  PartitionMemoryBudget=1024  PartitionMethod=ROBUST
      settings: SourceProductBaseCode=SS,PW,VE
  TL : fl_lib/Mechanical/Mechanical Sources/Ideal Torque Source
      settings: SourceProductBaseCode=PW,SS,VE
  "Tm " : fl_lib/Mechanical/Mechanical Sources/Ideal Torque Source
      settings: SourceProductBaseCode=PW,SS,VE
  mass spring mass : mass_spring_mass_lib/mass spring mass  b1=b N*m/(rad/s)  J1=J1 kg*m^2  b2=b N*m/(rad/s)  J2=J2 kg*m^2  b_theta=b_theta N*m/(rad/s)  k_theta=k_theta N*m/rad  omega_1_specify=off  omega_1_priority=None  omega_1=0 rad/s  omega_1_nominal_specify=off  omega_1_nominal_unit=rad/s  omega_1_nominal_value=1  omega_2_specify=off  omega_2_priority=None  omega_2=0 rad/s  omega_2_nominal_specify=off  omega_2_nominal_unit=rad/s  omega_2_nominal_value=1  tau_1_specify=off  tau_1_priority=None  tau_1=0 N*m  tau_1_nominal_specify=off  tau_1_nominal_unit=N*m  tau_1_nominal_value=1  tau_2_specify=off  tau_2_priority=None  tau_2=0 N*m  tau_2_nominal_specify=off  tau_2_nominal_unit=N*m  tau_2_nominal_value=1  tau_theta_specify=off  tau_theta_priority=None  tau_theta=0 N*m  tau_theta_nominal_specify=off  tau_theta_nominal_unit=N*m  tau_theta_nominal_value=1
      settings: InternalSimscapePortConfiguration="{\"Bottom\":[],\"Left\":[{\"id\":\"S1\",\"label\":\"S1\",\"type\":\"foundation.mechanical.rotational.rotational\"}],\"Right\":[{\"id\":\"S2\",\"label\":\"S2\",\"type\":\"foundation.mechanical.rotational.rotational\"},{\"id\":\"omega1_out\",\"label\":\"omega1\",\"type\":\"output\"},{\"id\":\"omega2_out\",\"label\":\"omega2\",\"type\":\"output\"},{\"id\":\"tau_theta_out\",\"label\":\"tau_theta\",\"type\":\"output\"}],\"Top\":[]}"
  w1 : Outport
  w2 : Outport  Port=2
  wires:
  PS-Simulink Converter3/1 -> w2/1
  Gain5/1 -> Simulink-PS Converter1/1
  tau1/1 -> [tau_1]
  [tau_1] -> Simulink-PS Converter2/1
  tau2/1 -> [tau_2]
  [tau_2] -> Gain5/1
  PS-Simulink Converter2/1 -> w1/1
  connections:
  Simulink-PS Converter2/RConn1 -- "Tm "/RConn1
  mass spring mass/LConn1 -- "Tm "/LConn1
  Simulink-PS Converter1/RConn1 -- TL/RConn1
  mass spring mass/RConn1 -- TL/LConn1
  Solver Configuration1/RConn1 -- "Tm "/RConn2 -- Mechanical Rotational Reference1/LConn1
  Mechanical Rotational Reference2/LConn1 -- TL/RConn2
  mass spring mass/RConn2 -- PS-Simulink Converter2/LConn1
  mass spring mass/RConn3 -- PS-Simulink Converter3/LConn1

== system mpc_inertia_mass/sf_ctrl/observer td ==
  u : Inport
  y : Inport  Port=2
  Gain1 : Gain  Gain=Lled  Multiplication=Matrix(K*u)
  Gain5 : Gain  Gain=Bled  Multiplication=Matrix(K*u)
  Gain6 : Gain  Gain=Cle  Multiplication=Matrix(K*u)
  Gain7 : Gain  Gain=Aled  Multiplication=Matrix(K*u)
  Sum1 : Sum  Inputs=|+-
  Sum2 : Sum  Inputs=++|
  Sum3 : Sum  Inputs=|++
  Unit Delay1 : UnitDelay  SampleTime=tcontrol  HasFrameUpgradeWarning=on
  x_hat : Outport
  y_hat : Outport  Port=2
  wires:
  Sum2/1 -> Sum3/1
  Sum3/1 -> Unit Delay1/1
  Gain7/1 -> Sum3/2
  Gain6/1 -> y_hat/1, Sum1/2
  Sum1/1 -> Gain1/1
  u/1 -> Gain5/1
  Gain1/1 -> Sum2/1
  Gain5/1 -> Sum2/2
  Unit Delay1/1 -> x_hat/1, Gain7/1, Gain6/1
  y/1 -> Sum1/1

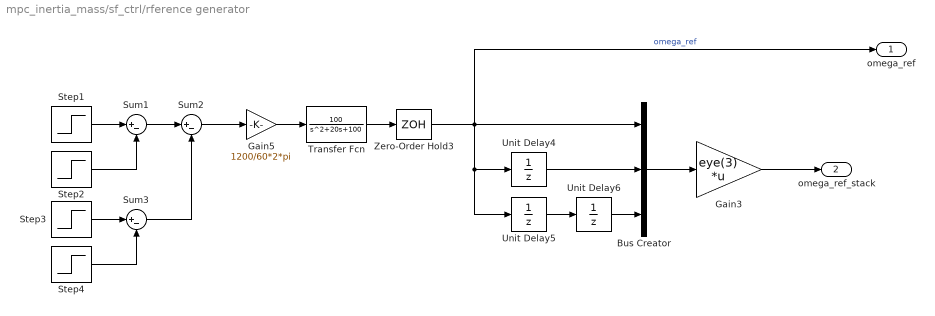
== system mpc_inertia_mass/sf_ctrl/rference generator ==
  Bus Creator : BusCreator  Inputs=3
  Gain3 : Gain  Gain=eye(3)  Multiplication=Matrix(K*u)
  Gain5 : Gain  Gain=1200/60*2*pi
  Step1 : Step  Time=2  SampleTime=0
  Step2 : Step  Time=simlength/4  SampleTime=0
  Step3 : Step  Time=simlength/2  SampleTime=0
  Step4 : Step  Time=2*simlength/3  SampleTime=0
  Sum1 : Sum  Inputs=|+-
  Sum2 : Sum  Inputs=|+-
  Sum3 : Sum  Inputs=|+-
  Transfer Fcn : TransferFcn  Numerator=[100]  Denominator=[1 20 100]
  Unit Delay4 : UnitDelay  SampleTime=tcontrol  HasFrameUpgradeWarning=on
  Unit Delay5 : UnitDelay  SampleTime=tcontrol  HasFrameUpgradeWarning=on
  Unit Delay6 : UnitDelay  SampleTime=tcontrol  HasFrameUpgradeWarning=on
  Zero-Order Hold3 : ZeroOrderHold  SampleTime=tcontrol
  omega_ref : Outport
  omega_ref_stack : Outport  Port=2
  wires:
  Unit Delay4/1 -> Bus Creator/2
  Sum2/1 -> Gain5/1
  Bus Creator/1 -> Gain3/1
  Zero-Order Hold3/1 -> omega_ref/1, Unit Delay4/1, Unit Delay5/1, Bus Creator/1  "omega_ref"
  Unit Delay6/1 -> Bus Creator/3
  Unit Delay5/1 -> Unit Delay6/1
  Step2/1 -> Sum1/2
  Transfer Fcn/1 -> Zero-Order Hold3/1
  Step1/1 -> Sum1/1
  Gain3/1 -> omega_ref_stack/1
  Sum1/1 -> Sum2/1
  Step3/1 -> Sum3/1
  Step4/1 -> Sum3/2
  Sum3/1 -> Sum2/2
  Gain5/1 -> Transfer Fcn/1
